simulink model "test"  (R2022b)
settings: Solver=VariableStepAuto  StartTime=0.0  StopTime=10.0  RelTol=1e-3
libraries: fl_lib x17, nesl_utility x5
settings Model: Creator=masam  LastModifiedBy=masam
settings SimscapeCC: SimscapeLogType=all  SimscapeLogSimulationStatistics=on  SimscapeLogName=simlog3  SimscapeLogDataHistory=15000

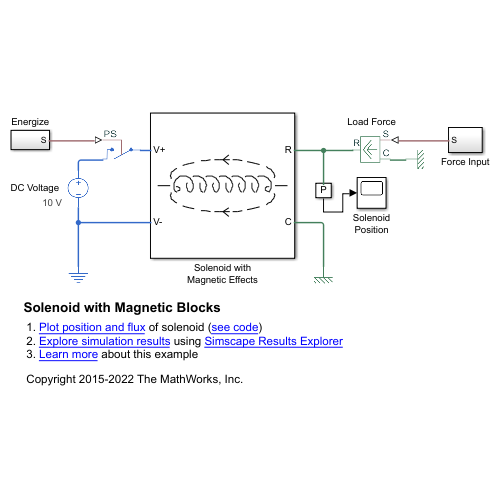
[thumbnail: Simulink's stored preview of the top-level diagram]
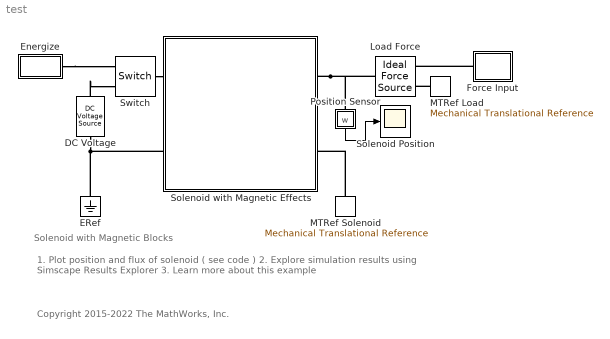
== system test ==
  note: 1. Plot position and flux of solenoid ( see code )
      | 2. Explore simulation results using Simscape Results Explorer
      | 3. Learn more about this example
  note: Copyright 2015-2022 The MathWorks, Inc.
  note: Solenoid with Magnetic Blocks
  DC Voltage : fl_lib/Electrical/Electrical Sources/DC Voltage Source  v0=10 V
      settings: AttributesFormatString=%<v0> %<v0_unit>
  ERef : fl_lib/Electrical/Electrical Elements/Electrical Reference
  Energize : Subsystem
  Force Input : Subsystem
  Load Force : fl_lib/Mechanical/Mechanical Sources/Ideal Force Source
  MTRef Load : fl_lib/Mechanical/Translational Elements/Mechanical Translational Reference
  MTRef Solenoid : fl_lib/Mechanical/Translational Elements/Mechanical Translational Reference
  Position Sensor : Subsystem
      mask Display: disp('P');
  Solenoid Position : Scope
  Solenoid with Magnetic Effects : Subsystem  Tag=PublishSubsystem
      mask Display:
      | % Solenoid coil (each turn two plot statements, last in one)
      | plot(sin(-1*pi/8:0.1:+3*pi/4)*0.15+0.6,cos(-1*pi/8:0.1:+3*pi/4)*0.15+0);
      | plot(sin(-3*pi/4:0.1:-3*pi/8)*0.15+0.6,cos(-3*pi/4:0.1:-3*pi/8)*0.15+0);
      | plot(sin(-1*pi/8:0.1:+3*pi/4)*0.15+0.4,cos(-1*pi/8:0.1:+3*pi/4)*0.15+0);
      | plot(sin(-3*pi/4:0.1:-3*pi/8)*0.15+0.4,cos(-3*pi/4:0.1:-3*pi/8)*0.15+0);
      | plot(sin(-1*pi/8:0.1:+3*pi/4)*0.15+0.2,cos(-1*pi/8:0.1:+3*pi/4)*0.15+0);
      | plot(sin(-3*pi/4:0.1:-3*pi/8)*0.15+0.2,cos(-3*pi/4:0.1:-3*pi/8)*0.15+0);
      | plot(sin(-1*pi/8:0.1:+3*pi/4)*0.15+0.0,cos(-1*pi/8:0.1:+3*pi/4)*0.15+0);
      | plot(sin(-3*pi/4:0.1:-3*pi/8)*0.15+0.0,cos(-3*pi/4:0.1:-3*pi/8)*0.15+0);
      | plot(sin(-1*pi/8:0.1:+3*pi/4)*0.15-0.2,cos(-1*pi/8:0.1:+3*pi/4)*0.15+0);
      | plot(sin(-3*pi/4:0.1:-3*pi/8)*0.15-0.2,cos(-3*pi/4:0.1:-3*pi/8)*0.15+0);
      | plot(sin(-1*pi/8:0.1:+3*pi/4)*0.15-0.4,cos(-1*pi/8:0.1:+3*pi/4)*0.15+0);
      | plot(sin(-3*pi/4:0.1:-3*pi/8)*0.15-0.4,cos(-3*pi/4:0.1:-3*pi/8)*0.15+0);
      | plot(sin(-3*pi/4:0.1:+3*pi/4)*0.15-0.6,cos(-3*pi/4:0.1:+3*pi/4)*0.15+0);
      | 
      | % Coil to wire
      | plot(sin(+1*pi/5:0.1:+3*pi/4)*0.15-0.8,cos(+1*pi/5:0.1:+3*pi/4)*0.05-0.05);
      | plot(sin(-13*pi/16:0.1:-3*pi/16)*0.15+0.8,cos(-13*pi/16:0.1:-3*pi/16)*0.05-0.05);
      | 
      | % Wire
      | plot([-1.0 -0.8],[0 0]);
      | plot([1.0 0.8],[0 0]);
      | 
      | % Magnetic field (upper, lower)
      | plot(sin(-9.0*pi/16:0.1:-5.0*pi/16)*0.8-0.0,cos(-9.0*pi/16:0.1:-5.0*pi/16)*0.25+0.15);
      | plot(sin(-4.5*pi/16:0.1:-2.5*pi/16)*0.8-0.0,cos(-4.5*pi/16:0.1:-2.5*pi/16)*0.25+0.15);
      | plot(sin(-2.2*pi/16:0.1:-0.9*pi/16)*0.8-0.0,cos(-2.2*pi/16:0.1:-0.9*pi/16)*0.25+0.15);
      | plot(sin(-0.8*pi/16:0.1:+0.8*pi/16)*0.8-0.0,cos(-0.8*pi/16:0.1:+0.8*pi/16)*0.25+0.15);
      | plot(sin(+1.0*pi/16:0.1:+2.2*pi/16)*0.8-0.0,cos(+1.0*pi/16:0.1:+2.2*pi/16)*0.25+0.15);
      | plot(sin(+2.5*pi/16:0.1:+4.5*pi/16)*0.8-0.0,cos(+2.5*pi/16:0.1:+4.5*pi/16)*0.25+0.15);
      | plot(sin(+5.0*pi/16:0.1:+9.0*pi/16)*0.8-0.0,cos(+5.0*pi/16:0.1:+9.0*pi/16)*0.25+0.15);
      | plot([0 0.1],[0.4 0.47]);
      | plot([0 0.1],[0.4 0.33]);
      | 
      | plot(sin(-9.0*pi/16:0.1:-5.0*pi/16)*0.8-0.0,-cos(-9.0*pi/16:0.1:-5.0*pi/16)*0.25-0.15);
      | plot(sin(-4.5*pi/16:0.1:-2.5*pi/16)*0.8-0.0,-cos(-4.5*pi/16:0.1:-2.5*pi/16)*0.25-0.15);
      | plot(sin(-2.2*pi/16:0.1:-0.9*pi/16)*0.8-0.0,-cos(-2.2*pi/16:0.1:-0.9*pi/16)*0.25-0.15);
      | plot(sin(-0.8*pi/16:0.1:+0.8*pi/16)*0.8-0.0,-cos(-0.8*pi/16:0.1:+0.8*pi/16)*0.25-0.15);
      | plot(sin(+1.0*pi/16:0.1:+2.2*pi/16)*0.8-0.0,-cos(+1.0*pi/16:0.1:+2.2*pi/16)*0.25-0.15);
      | plot(sin(+2.5*pi/16:0.1:+4.5*pi/16)*0.8-0.0,-cos(+2.5*pi/16:0.1:+4.5*pi/16)*0.25-0.15);
      | plot(sin(+5.0*pi/16:0.1:+9.0*pi/16)*0.8-0.0,-cos(+5.0*pi/16:0.1:+9.0*pi/16)*0.25-0.15);
      | plot([0 0.1],-[0.4 0.47]);
      | plot([0 0.1],-[0.4 0.33]);
      | 
      | 
      | % Plot points to set plot range
      | color('white');plot(1.1,1.1);plot(-1.1,-1.1)
      | color('black');
      | 
      | port_label('RConn',1,'R');
      | port_label('RConn',2,'C');
      | port_label('LConn',1,'V+');
      | port_label('LConn',2,'V-');
  Switch : fl_lib/Electrical/Electrical Elements/Switch  R_closed=0.01 Ohm  G_open=1e-08 1/Ohm  Threshold=0  i_specify=off  i_priority=High  i=0 A  i_nominal_specify=off  i_nominal_unit=A  i_nominal_value=1  v_specify=off  v_priority=High  v=0 V  v_nominal_specify=off  v_nominal_unit=V  v_nominal_value=1
  wires:
  Position Sensor/1(w) -> Solenoid Position/1
  connections:
  Solenoid with Magnetic Effects/RConn1 -- Load Force/LConn1 -- Position Sensor/LConn1
  DC Voltage/RConn1 -- Solenoid with Magnetic Effects/LConn2 -- ERef/LConn1
  Force Input/LConn1 -- Load Force/RConn1
  Energize/RConn1 -- Switch/RConn1
  Switch/LConn1 -- Solenoid with Magnetic Effects/LConn1
  MTRef Solenoid/LConn1 -- Solenoid with Magnetic Effects/RConn2
  MTRef Load/LConn1 -- Load Force/RConn2
  DC Voltage/LConn1 -- Switch/RConn2

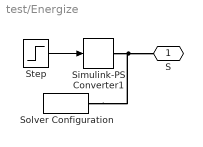
== system test/Energize ==
  Simulink-PS Converter1 : nesl_utility/Simulink-PS Converter  PhysicalDomain=network_engine_domain  SubClassName=ps_input  LeftPortType=input  RightPortType=output  PseudoPeriodic=off  Frequencies=[]  NoiseDistribution=none  NoiseParameters=[]  Unit=1  AffineConversion=off  FilteringAndDerivatives=zero  SimscapeFilterOrder=1  InputFilterTimeConstant=.001  UdotUserProvided=0
  Solver Configuration : nesl_utility/Solver Configuration  PhysicalDomain=network_engine_domain  SubClassName=solver  LeftPortType=input  RightPortType=generic  Tones=[]  Harmonics=[]  SimulateNoise=off  Profile=off  UseLocalSampling=off  EnableSwitchedLinearOptims=on  FrequencyDomain=off  UseCCode=off  RelTol=0.001  AbsTol=1e-06  MinStep=1e-09  ToWorkspace=off  RevertToSquareIcSolve=off  NumHomotopyIterations=100  PhasorMode=off  PhasorModeNumHarmonics=1  ConsistencySolver=NEWTON_XTOL_AFTER_FTOL  IndexReductionMethod=DerivativeReplacement  DoDC=off  ResidualTolerance=1e-9  ConsistencyTolSource=GLOBAL  ConsistencyAbsTol=0.001  ConsistencyRelTol=0.001  ConsistencyTolFactor=0.001  UseLocalSolver=off  LocalSolverChoice=NE_BACKWARD_EULER_ADVANCER  ResolveIndetEquations=on  FunctionEvalNumThread=1  LocalSolverSampleTime=.001  DoFixedCost=off  MaxNonlinIter=3  MaxModeIter=2  ComputeImpulses=off  ImpulseIterations=2  LinearAlgebra=auto  LinearAlgebraNumThread=0  EquationFormulation=NE_TIME_EF  DelaysMemoryBudget=1024  AutomaticFiltering=on  FilteringTimeConstant=0.001  PartitionStorageMethod=AS_NEEDED  PartitionMemoryBudget=1024  PartitionMethod=FAST
  Step : Step  Time=0.1  SampleTime=0
  S : PMIOPort  Side=Right
  wires:
  Step/1 -> Simulink-PS Converter1/1
  connections:
  Simulink-PS Converter1/RConn1 -- Solver Configuration/RConn1 -- S/RConn1

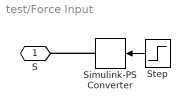
== system test/Force Input ==
  Simulink-PS Converter : nesl_utility/Simulink-PS Converter  PhysicalDomain=network_engine_domain  SubClassName=ps_input  LeftPortType=input  RightPortType=output  PseudoPeriodic=off  Frequencies=[]  NoiseDistribution=none  NoiseParameters=[]  Unit=1  AffineConversion=off  FilteringAndDerivatives=zero  SimscapeFilterOrder=1  InputFilterTimeConstant=.001  UdotUserProvided=0
  Step : Step  Time=0.3  After=10  SampleTime=0
  S : PMIOPort  Side=Left
  wires:
  Step/1 -> Simulink-PS Converter/1
  connections:
  Simulink-PS Converter/RConn1 -- S/RConn1

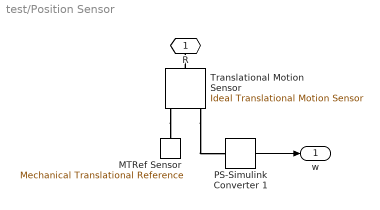
== system test/Position Sensor ==
  MTRef Sensor : fl_lib/Mechanical/Translational Elements/Mechanical Translational Reference
  PS-Simulink Converter 1 : nesl_utility/PS-Simulink Converter  PhysicalDomain=network_engine_domain  SubClassName=ps_output  LeftPortType=input  RightPortType=output  PseudoPeriodic=off  Frequencies=[]  VectorFormat=1-D array  Unit=mm  AffineConversion=off
  Translational Motion Sensor : fl_lib/Mechanical/Mechanical Sensors/Ideal Translational Motion Sensor  reference=foundation.enum.MeasurementReference.difference  acceleration_port=false  velocity_port=true  position_port=true  offset=5 mm
  R : PMIOPort  Side=Left
  w : Outport  VectorParamsAs1DForOutWhenUnconnected=off
  wires:
  PS-Simulink Converter 1/1 -> w/1
  connections:
  Translational Motion Sensor/LConn1 -- R/RConn1
  Translational Motion Sensor/RConn1 -- MTRef Sensor/LConn1
  Translational Motion Sensor/RConn3 -- PS-Simulink Converter 1/LConn1

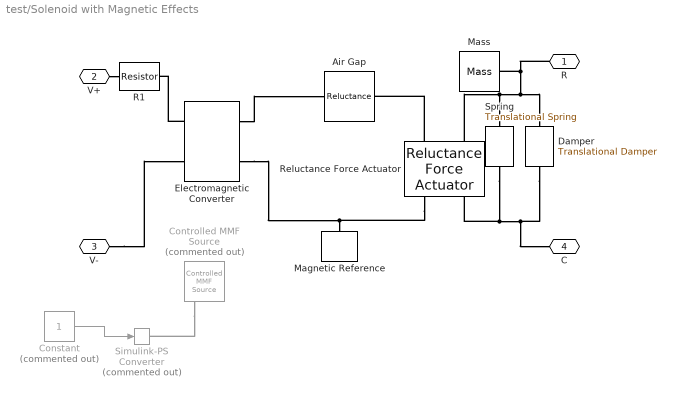
== system test/Solenoid with Magnetic Effects ==
  " Air Gap" : fl_lib/Magnetic/Magnetic Elements/Reluctance  g=1 mm  CSA=4 cm^2  mur=1  phi_specify=off  phi_priority=High  phi=0 Wb  phi_nominal_specify=off  phi_nominal_unit=Wb  phi_nominal_value=1  mmf_specify=off  mmf_priority=High  mmf=0 A  mmf_nominal_specify=off  mmf_nominal_unit=A  mmf_nominal_value=1
      settings: InternalSimscapePortConfiguration="{\"Bottom\":[],\"Left\":[{\"id\":\"N\",\"label\":\"N\",\"type\":\"foundation.magnetic.magnetic\"}],\"Right\":[{\"id\":\"S\",\"label\":\"S\",\"type\":\"foundation.magnetic.magnetic\"}],\"Top\":[]}"
  Constant : Constant  Commented=on
  Controlled MMF Source : fl_lib/Magnetic/Magnetic Sources/Controlled MMF Source  Commented=on
      settings: InternalSimscapePortConfiguration="{\"Bottom\":[],\"Left\":[{\"id\":\"N\",\"label\":\"\",\"type\":\"foundation.magnetic.magnetic\"}],\"Right\":[{\"id\":\"mmfI\",\"label\":\"\",\"type\":\"input\"},{\"id\":\"S\",\"label\":\"\",\"type\":\"foundation.magnetic.magnetic\"}],\"Top\":[]}"
  Damper : fl_lib/Mechanical/Translational Elements/Translational Damper  D=20 N/(m/s)  v_specify=off  v_priority=High  v=0 m/s  v_nominal_specify=off  v_nominal_unit=m/s  v_nominal_value=1  f_specify=off  f_priority=High  f=0 N  f_nominal_specify=off  f_nominal_unit=N  f_nominal_value=1
  Electromagnetic Converter : fl_lib/Magnetic/Magnetic Elements/Electromagnetic Converter  Nw=17  i_specify=off  i_priority=High  i=0 A  i_nominal_specify=off  i_nominal_unit=A  i_nominal_value=1  v_specify=off  v_priority=High  v=0 V  v_nominal_specify=off  v_nominal_unit=V  v_nominal_value=1  mmf_specify=off  mmf_priority=High  mmf=0 A  mmf_nominal_specify=off  mmf_nominal_unit=A  mmf_nominal_value=1  phi_specify=off  phi_priority=High  phi=0 Wb  phi_nominal_specify=off  phi_nominal_unit=Wb  phi_nominal_value=1
      settings: InternalSimscapePortConfiguration="{\"Bottom\":[],\"Left\":[{\"id\":\"p\",\"label\":\"+\",\"type\":\"foundation.electrical.electrical\"},{\"id\":\"n\",\"label\":\"-\",\"type\":\"foundation.electrical.electrical\"}],\"Right\":[{\"id\":\"N\",\"label\":\"N\",\"type\":\"foundation.magnetic.magnetic\"},{\"id\":\"S\",\"label\":\"S\",\"type\":\"foundation.magnetic.magnetic\"}],\"Top\":[]}"
  Magnetic Reference : fl_lib/Magnetic/Magnetic Elements/Magnetic Reference
      settings: InternalSimscapePortConfiguration="{\"Bottom\":[],\"Left\":[{\"id\":\"M\",\"label\":\"\",\"type\":\"foundation.magnetic.magnetic\"}],\"Right\":[],\"Top\":[]}"
  Mass : fl_lib/Mechanical/Translational Elements/Mass  mass=0.1 kg  num_ports=foundation.enum.numPorts2.one  v_specify=off  v_priority=High  v=0 m/s  v_nominal_specify=off  v_nominal_unit=m/s  v_nominal_value=1  f_specify=off  f_priority=High  f=0 N  f_nominal_specify=off  f_nominal_unit=N  f_nominal_value=1
  R1 : fl_lib/Electrical/Electrical Elements/Resistor  R=10 Ohm  i_specify=off  i_priority=High  i=0 A  i_nominal_specify=off  i_nominal_unit=A  i_nominal_value=1  v_specify=off  v_priority=High  v=0 V  v_nominal_specify=off  v_nominal_unit=V  v_nominal_value=1
  Reluctance Force Actuator : fl_lib/Magnetic/Magnetic Elements/Reluctance Force Actuator  x0=5 mm  xmin=1e-9 mm  CSA=4 cm^2  mur=1  K_contact=1e6 N/m  D_contact=50 N/(m/s)  mmf_specify=off  mmf_priority=High  mmf=0 A  mmf_nominal_specify=off  mmf_nominal_unit=A  mmf_nominal_value=1  phi_specify=off  phi_priority=High  phi=0 Wb  phi_nominal_specify=off  phi_nominal_unit=Wb  phi_nominal_value=1  f_specify=off  f_priority=High  f=0 N  f_nominal_specify=off  f_nominal_unit=N  f_nominal_value=1  u_specify=off  u_priority=High  u=0 m/s  u_nominal_specify=off  u_nominal_unit=m/s  u_nominal_value=1
      settings: InternalSimscapePortConfiguration="{\"Bottom\":[],\"Left\":[{\"id\":\"N\",\"label\":\"N\",\"type\":\"foundation.magnetic.magnetic\"},{\"id\":\"R\",\"label\":\"R\",\"type\":\"foundation.mechanical.translational.translational\"}],\"Right\":[{\"id\":\"S\",\"label\":\"S\",\"type\":\"foundation.magnetic.magnetic\"},{\"id\":\"C\",\"label\":\"C\",\"type\":\"foundation.mechanical.translational.translational\"}],\"Top\":[]}"
  Simulink-PS Converter : nesl_utility/Simulink-PS Converter  Commented=on  PhysicalDomain=network_engine_domain  SubClassName=ps_input  LeftPortType=input  RightPortType=output  PseudoPeriodic=off  Frequencies=[]  NoiseDistribution=none  NoiseParameters=[]  Unit=1  AffineConversion=off  FilteringAndDerivatives=provide  SimscapeFilterOrder=1  InputFilterTimeConstant=0.001  UdotUserProvided=0
  Spring : fl_lib/Mechanical/Translational Elements/Translational Spring  spr_rate=200 N/m  v_specify=off  v_priority=High  v=0 m/s  v_nominal_specify=off  v_nominal_unit=m/s  v_nominal_value=1  f_specify=off  f_priority=High  f=0 N  f_nominal_specify=off  f_nominal_unit=N  f_nominal_value=1  x_specify=off  x_priority=High  x=0 mm  x_nominal_specify=off  x_nominal_unit=m  x_nominal_value=1
  R : PMIOPort  Side=Right
  V+ : PMIOPort  Port=2  Side=Left
  V- : PMIOPort  Port=3  Side=Left
  C : PMIOPort  Port=4  Side=Right
  wires:
  Constant/1 -> Simulink-PS Converter/1
  connections:
  V-/RConn1 -- Electromagnetic Converter/LConn2
  Electromagnetic Converter/LConn1 -- R1/RConn1
  V+/RConn1 -- R1/LConn1
  Mass/LConn1 -- Damper/LConn1 -- Reluctance Force Actuator/LConn2 -- Spring/LConn1 -- R/RConn1
  Reluctance Force Actuator/RConn2 -- Damper/RConn1 -- C/RConn1 -- Spring/RConn1
  Electromagnetic Converter/RConn1 -- " Air Gap"/LConn1
  Reluctance Force Actuator/LConn1 -- " Air Gap"/RConn1
  Reluctance Force Actuator/RConn1 -- Electromagnetic Converter/RConn2 -- Magnetic Reference/LConn1
  Controlled MMF Source/RConn1 -- Simulink-PS Converter/RConn1
